simulink model "hw2S"  (R2014b)
settings: Solver=ode3  StartTime=0.0  StopTime=10.0  FixedStep=1/(fs)  RelTol=1e-3
values from neighbouring files (symbols this model uses):
  den = sym2poly(den)    [hw2.m]
  fs = 2000    [hw2.m]
  input_selector = 2    [hw2.m]
  num = sym2poly(num)    [hw2.m]
settings Model: Creator=lq561d  LastModifiedBy=lq561d

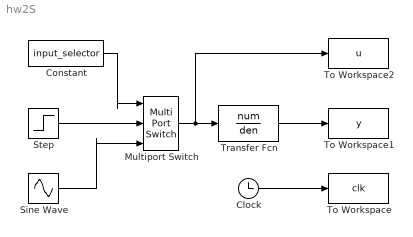
== system hw2S ==
  Clock : Clock
  Constant : Constant  Value=input_selector
  Multiport Switch : MultiPortSwitch  Inputs=2
  Sine Wave : Sin  Bias=-1  Frequency=1000  SampleTime=1/fs
  Step : Step  Time=0  SampleTime=0
  To Workspace : ToWorkspace  VariableName=clk  SampleTime=-1
  To Workspace1 : ToWorkspace  VariableName=y  SampleTime=-1
  To Workspace2 : ToWorkspace  VariableName=u  SampleTime=-1
  Transfer Fcn : TransferFcn  Numerator=num  Denominator=den
  wires:
  Clock/1 -> To Workspace/1
  Transfer Fcn/1 -> To Workspace1/1
  Multiport Switch/1 -> To Workspace2/1, Transfer Fcn/1
  Constant/1 -> Multiport Switch/1
  Step/1 -> Multiport Switch/2
  Sine Wave/1 -> Multiport Switch/3
